simulink model "quadcopter_swarm_Perron"  (R2023b)
settings: Solver=ode3  StartTime=0  StopTime=inf  FixedStep=0.005  RelTol=1e-3  EnableMultiTasking=on
values from neighbouring files (symbols this model uses):
  F_e_g = [0 0 39.28]    [1nrx_dot.mat]    (also in 1nrxdrones_dot.mat; collision_avoidance_POS.mat; collision_avoidance_headonfix_POS.mat; collision_test.mat)
  g = 9.82    [1nrx_dot.mat]    (also in 1nrxdrones_dot.mat; collision_avoidance_POS.mat; collision_avoidance_headonfix_POS.mat; collision_test.mat)
  I_C = [0.5  0  0; 0  0.5  0; 0  0  1]    [1nrx_dot.mat]    (also in 1nrxdrones_dot.mat; collision_avoidance_POS.mat; collision_avoidance_headonfix_POS.mat; collision_test.mat)
  L = [4 -1 -1 -1 -1 0 -1 4 -1 -1 -1 0 ... (36 elements, 6x6)]    [1nrx_dot.mat]    (also in 1nrxdrones_dot.mat; collision_avoidance_POS.mat; collision_avoidance_headonfix_POS.mat; collision_test.mat)
  m = 4    [1nrx_dot.mat]    (also in 1nrxdrones_dot.mat; collision_avoidance_POS.mat; collision_avoidance_headonfix_POS.mat; collision_test.mat)
  M_RB = [4 0 0 0 0 0 0 4 0 0 0 0 ... (36 elements, 6x6)]    [1nrx_dot.mat]    (also in 1nrxdrones_dot.mat; collision_avoidance_POS.mat; collision_avoidance_headonfix_POS.mat; collision_test.mat)
  PID_inner_max = 100    [quadcopter_swarm_par.m]
  PID_outer_max = 10    [quadcopter_swarm_par.m]
  x_0 = [0, 3, 2, 1]'    [quadcopter_swarm_par.m]
  x_d = [1,4,-2,7]'    [quadcopter_swarm_par.m]
libraries: slpidlib x24, simulink_extras x20, dspsigops x12, aerolibutil x8, sharedtransform x4, vrlib x1
(part 1 of 5)
settings Model: Creator=The MathWorks, Inc.  LastModifiedBy=frank
settings SolverCC: AlgebraicLoopSolver=TrustRegion
settings DataIOCC: LimitDataPoints=on  SaveFormat=Array  SaveOutput=off  SignalLogging=off  DSMLogging=off  SaveTime=off  ReturnWorkspaceOutputs=off
settings OptimizationCC: BlockReduction=off  BufferReuse=off  LifeSpan=inf
settings DebuggingCC: AlgebraicLoopMsg=none  ParameterPrecisionLossMsg=none  AllowSymbolicDim=off  PregeneratedLibrarySubsystemCodeDiagnostic=none  SFUnexpectedBacktrackingDiag=warning  SFNoUnconditionalDefaultTransitionDiag=warning  SFExecutionAtInitializationDiag=none  ArithmeticOperatorsInVariantConditions=warning
settings HardwareCC: ProdBitPerPointer=32  ProdBitPerSizeT=32  ProdBitPerPtrDiffT=32  ProdLargestAtomicFloat=None  ProdIntDivRoundTo=Undefined  ProdEndianess=Unspecified  ProdWordSize=32  ProdHWDeviceType=32-bit Generic
settings ModelReferenceCC: EnableRefExpFcnMdlSchedulingChecks=on  PropagateSignalLabelsOutOfModel=off
settings SFSimCC: SimUseLocalCustomCode=off  CustomCodeUndefinedFunction=UseInterfaceOnly
settings RTWCC: RTWUseLocalCustomCode=off  DLArmComputeVersion=19.05
settings CodeAppCC: StateflowObjectComments=on
settings GRTTargetCC: TargetLangStandard=C89/C90 (ANSI)
settings ConfigComp: CovMetricSettings=dw  CovSaveCumulativeToWorkspaceVar=on  CovSaveSingleToWorkspaceVar=on  CovExternalEMLEnable=off  CovSFcnEnable=off

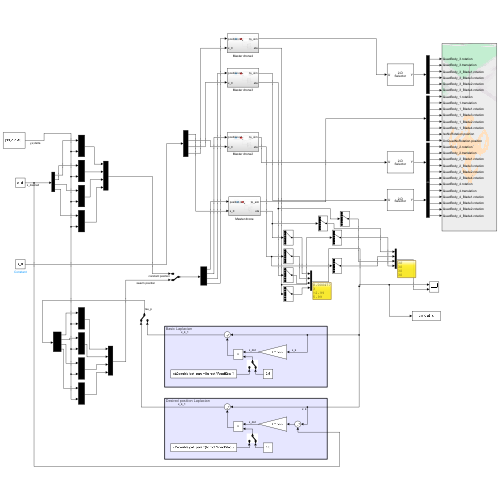
[thumbnail: Simulink's stored preview of the top-level diagram]
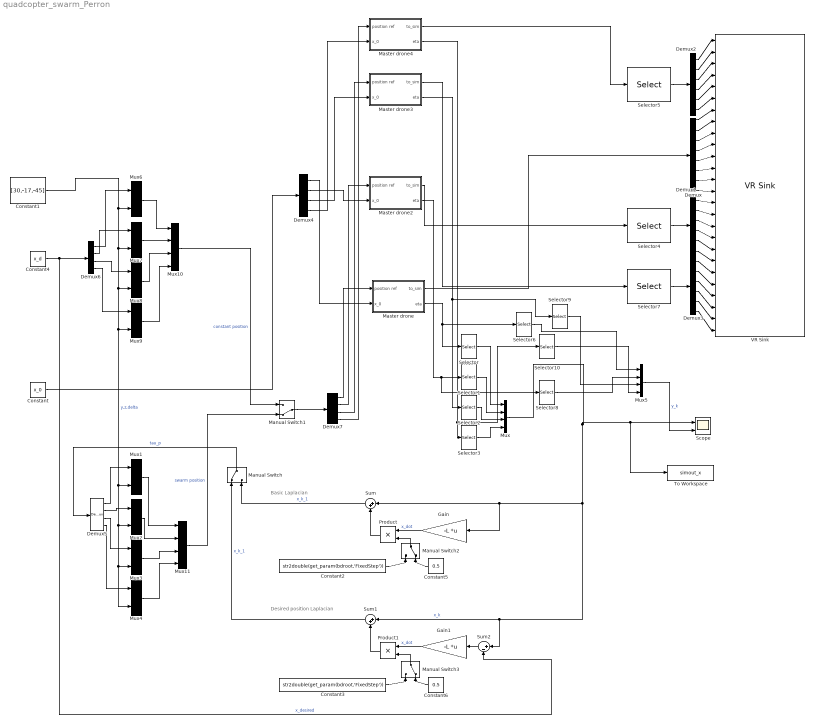
== system quadcopter_swarm_Perron ==
  note: Basic Laplacian
  note: Desired position Laplacian
  Constant : Constant  Value=x_0
  Constant1 : Constant  Value=[30,-17,-45]
  Constant2 : Constant  Value=str2double(get_param(bdroot,'FixedStep'))
  Constant3 : Constant  Value=str2double(get_param(bdroot,'FixedStep'))
  Constant4 : Constant  Value=x_d
  Constant5 : Constant  Value=0.5
  Constant6 : Constant  Value=0.5
  Demux : Demux  Outputs=8
  Demux1 : Demux  Outputs=6
  Demux2 : Demux  Outputs=6
  Demux3 : Demux  Outputs=6
  Demux{4..7} (4 alike) : Demux
  Gain : Gain  Gain=-L  Multiplication=Matrix(K*u) (u vector)
  Gain1 : Gain  Gain=-L  Multiplication=Matrix(K*u) (u vector)
  Manual Switch : ManualSwitch
  Manual Switch1 : ManualSwitch  CurrentSetting=0
  Manual Switch2 : ManualSwitch  CurrentSetting=0
  Manual Switch3 : ManualSwitch  CurrentSetting=0
  Master drone : Subsystem
  Master drone2 : Subsystem
  Master drone3 : Subsystem
  Master drone4 : Subsystem
  Mux{,5,10..11} (4 alike) : Mux
  Mux{1..4,6..9} (8 alike) : Mux  Inputs=2
  Product : Product
  Product1 : Product
  Scope : Scope  NumInputPorts=2
  Selector{,1..3} (4 alike) : Selector  InputPortWidth=6  IndexOptions=Index vector (dialog)  Indices=1  OutputSizes=1
  Selector{6,8..10} (4 alike) : Selector  InputPortWidth=6  IndexOptions=Index vector (dialog)  Indices=2  OutputSizes=1
  Selector4 : Selector  NumberOfDimensions=2  InputPortWidth=8  IndexOptions=Index vector (dialog),Select all  Indices=1:23,1  OutputSizes=1,1
  Selector5 : Selector  NumberOfDimensions=2  InputPortWidth=8  IndexOptions=Index vector (dialog),Select all  Indices=1:23,1  OutputSizes=1,1
  Selector7 : Selector  NumberOfDimensions=2  InputPortWidth=8  IndexOptions=Index vector (dialog),Select all  Indices=1:23,1  OutputSizes=1,1
  Sum : Sum  Inputs=|++
  Sum1 : Sum  Inputs=|++
  Sum2 : Sum  Inputs=|+-
  To Workspace : ToWorkspace  VariableName=simout_x  SampleTime=-1
      settings: Save2DSignal=2-D array (concatenate along first dimension)
  VR Sink : vrlib/VR Sink  InstantiateOnLoad=on  SampleTime=12*0.005  ViewEnable=on  RemoteChange=off  RemoteView=off  FieldsWritten=QuadBody_3.rotation.4.1.1.double#QuadBody_3.translation.3.1.1.double#QuadBody_3_Blade1.rotation.4.1.1.double#QuadBody_3_Blade3.rotation.4.1.1.double#QuadBody_3_Blade2.rotation.4.1.1.double#QuadBody_3_Blade4.rotation.4.1.1.double#QuadBody_1.rotation.4.1.1.double#QuadBody_1.translation.3.1.1.double#QuadBody_1_Blade1.rotation.4.1.1.double#QuadBody_1_Blade3.rotation.4.1.1.double#QuadBody_1_Blade2.rotation.4.1.1.double#QuadBody_1_Blade4.rotation.4.1.1.double#IsoNoRotation.position.3.1.1.double#OnQuadNoRotation.position.3.1.1.double#QuadBody_2.rotation.4.1.1.double#QuadBody_2.translation.3.1.1.double#QuadBody_2_Blade1.rotation.4.1.1.double#QuadBody_2_Blade3.rotation.4.1.1.double#QuadBody_2_Blade2.rotation.4.1.1.double#QuadBody_2_Blade4.rotation.4.1.1.double#QuadBody_4.rotation.4.1.1.double#QuadBody_4.translation.3.1.1.double#QuadBody_4_Blade1.rotation.4.1.1.double#QuadBody_4_Blade3.rotation.4.1.1.double#QuadBody_4_Blade2.rotation.4.1.1.double#QuadBody_4_Blade4.rotation.4.1.1.double  WorldFileName=Quadcopter_VR.wrl  AutoView=on  VideoDimensions=[]  AllowVariableSize=off  FigureProperties="{'Position', 'Name', 'Viewpoint', 'CameraBound', 'CameraDirection', 'CameraPosition', 'CameraUpVector', 'ZoomFactor', 'Antialiasing', 'Headlight', 'Lighting', 'NavPanel', 'Sound', 'StatusBar', 'Stereo3D', 'Stereo3DCameraOffset', 'Stereo3DHIT', 'ToolBar', 'Textures', 'Transparency', 'Triad', 'Wireframe', 'NavZones', 'NavMode', 'NavSpeed', 'CaptureFileFormat', 'CaptureFileName', 'Record2DCompressMethod', 'Record2DCompressQuality', 'Record2D', 'Record2DFileName', 'Record2DFPS'; [4.4020000000000000e+03   4.4400000000000000e+02   9.5800000000000000e+02   9.0400000000000000e+02], '', 'Isometric - No Rotation', 'on', [6.2775029607530120e-02  -3.1395260637159403e-02  -9.9753377550201194e-01], [0.0000000000000000e+00   0.0000000000000000e+00   1.5000000000000000e+01], [9.8663584075743787e-04   9.9950656033827134e-01  -3.1395260637159403e-02], [1.0000000000000000e+00], 'on', 'on', 'on', 'halfbar', 'on', 'on', 'off', [1.0000000149011612e-01], [0.0000000000000000e+00], 'on', 'on', 'on', 'none', 'off', 'off', 'fly', 'normal', 'tif', '%f_anim_%n.tif', 'auto', [7.5000000000000000e+01], 'off', '%f_anim_%n.avi', 'auto'}"
  wires:
  Demux/1 -> VR Sink/7
  Demux/2 -> VR Sink/8
  Demux/3 -> VR Sink/9
  Demux/4 -> VR Sink/10
  Demux/5 -> VR Sink/11
  Demux/6 -> VR Sink/12
  Demux1/1 -> VR Sink/15
  Demux1/2 -> VR Sink/16
  Demux1/3 -> VR Sink/17
  Demux1/4 -> VR Sink/18
  Demux1/5 -> VR Sink/19
  Demux1/6 -> VR Sink/20
  Demux3/1 -> VR Sink/21
  Demux3/2 -> VR Sink/22
  Demux3/3 -> VR Sink/23
  Demux3/4 -> VR Sink/24
  Demux3/5 -> VR Sink/25
  Demux3/6 -> VR Sink/26
  Demux2/6 -> VR Sink/6
  Demux2/5 -> VR Sink/5
  Demux2/4 -> VR Sink/4
  Demux2/3 -> VR Sink/3
  Demux2/2 -> VR Sink/2
  Demux2/1 -> VR Sink/1
  Selector5/1 -> Demux2/1
  Selector7/1 -> Demux3/1
  Master drone4/1(to_sim) -> Selector5/1
  Selector4/1 -> Demux1/1
  Demux/7 -> VR Sink/13
  Demux/8 -> VR Sink/14
  Master drone/1(to_sim) -> Demux/1
  Master drone2/1(to_sim) -> Selector4/1
  Master drone3/1(to_sim) -> Selector7/1
  Master drone/2(eta) -> Selector/1, Selector6/1
  Master drone2/2(eta) -> Selector8/1, Selector1/1
  Master drone3/2(eta) -> Selector2/1, Selector9/1
  Master drone4/2(eta) -> Selector3/1, Selector10/1
  Selector/1 -> Mux/1
  Selector1/1 -> Mux/2
  Selector2/1 -> Mux/3
  Selector3/1 -> Mux/4
  Constant/1 -> Demux4/1
  Demux4/1 -> Master drone/2(x_0)
  Demux4/2 -> Master drone2/2(x_0)
  Demux4/3 -> Master drone3/2(x_0)
  Demux4/4 -> Master drone4/2(x_0)
  Sum/1 -> Manual Switch/2  "x_k_1"
  Demux7/1 -> Master drone/1(position ref)
  Demux5/1 -> Mux1/1
  Demux5/2 -> Mux2/1
  Demux7/2 -> Master drone2/1(position ref)
  Demux5/3 -> Mux3/1
  Demux5/4 -> Mux4/1
  Demux7/3 -> Master drone3/1(position ref)
  Demux7/4 -> Master drone4/1(position ref)
  Selector6/1 -> Mux5/1
  Selector8/1 -> Mux5/2
  Selector9/1 -> Mux5/3
  Selector10/1 -> Mux5/4
  Mux5/1 -> Scope/2  "y_k"
  Gain/1 -> Product/1  "x_dot"
  Constant2/1 -> Manual Switch2/1
  Product/1 -> Sum/2
  Product1/1 -> Sum1/2
  Sum1/1 -> Manual Switch/1  "x_k_1"
  Gain1/1 -> Product1/1  "x_dot"
  Mux/1 -> Sum2/1, Sum1/1, Sum/1, Gain/1, To Workspace/1, Scope/1  "x_k"
  Manual Switch/1 -> Demux5/1  "tau_p"
  Constant1/1 -> Mux4/2, Mux3/2, Mux2/2, Mux1/2, Mux9/2, Mux8/2, Mux7/2, Mux6/2  "y,z,delta"
  Mux6/1 -> Mux10/1
  Mux7/1 -> Mux10/2
  Mux8/1 -> Mux10/3
  Mux9/1 -> Mux10/4
  Manual Switch1/1 -> Demux7/1
  Mux11/1 -> Manual Switch1/2  "swarm position"
  Mux10/1 -> Manual Switch1/1  "constant position"
  Mux1/1 -> Mux11/1
  Mux2/1 -> Mux11/2
  Mux3/1 -> Mux11/3
  Mux4/1 -> Mux11/4
  Constant4/1 -> Sum2/2, Demux6/1  "x_desired"
  Demux6/1 -> Mux6/1
  Demux6/2 -> Mux7/1
  Demux6/3 -> Mux8/1
  Demux6/4 -> Mux9/1
  Constant5/1 -> Manual Switch2/2
  Manual Switch2/1 -> Product/2
  Sum2/1 -> Gain1/1
  Constant6/1 -> Manual Switch3/2
  Constant3/1 -> Manual Switch3/1
  Manual Switch3/1 -> Product1/2

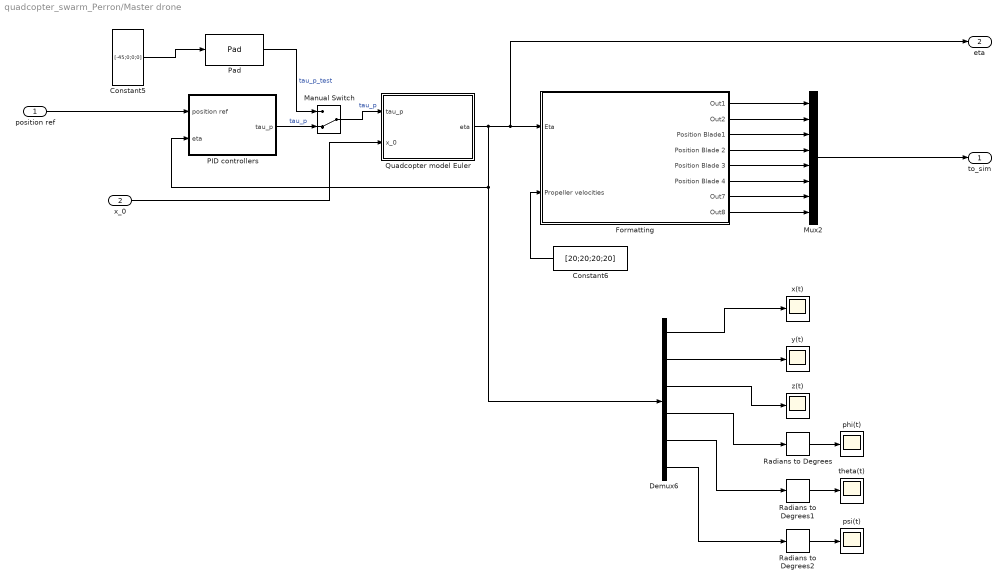
== system quadcopter_swarm_Perron/Master drone ==
  position ref : Inport
  x_0 : Inport  Port=2
  Constant5 : Constant  Value=[-45;0;0;0]  VectorParams1D=off
  Constant6 : Constant  Value=[20;20;20;20]  VectorParams1D=off
  Demux6 : Demux  Outputs=6
  Formatting : Subsystem
  Manual Switch : ManualSwitch  CurrentSetting=0
  Mux2 : Mux  Inputs=8
  PID controllers : Subsystem
  Pad : dspsigops/Pad  padAlong=Specified dimensions  dimsToPad=1  valSrc=Specify via dialog  padVal=0  spec=Output size  padNumOutRowsSpecMethod=User-specified  numOutRows=1  padNumOutColsSpecMethod=User-specified  numOutCols=6  isVarDimsMode=off  padBeginning=0  padEnd=0  outSizeMode=User-specified  outSize=6  padSigAt=Beginning  trunc_flag=None  roundingMode=Floor  overflowMode=off  truncOrWrapMode=Truncate  wrap_flag=None
  Quadcopter model Euler : Subsystem
  Radians to Degrees : simulink_extras/Transformations/Radians to Degrees
  Radians to Degrees1 : simulink_extras/Transformations/Radians to Degrees
  Radians to Degrees2 : simulink_extras/Transformations/Radians to Degrees
  phi(t) : Scope
  psi(t) : Scope
  theta(t) : Scope
  x(t) : Scope
  y(t) : Scope
  z(t) : Scope
  to_sim : Outport
  eta : Outport  Port=2
  wires:
  Formatting/6(Position Blade 4) -> Mux2/6
  Demux6/1 -> x(t)/1
  Demux6/6 -> Radians to Degrees2/1
  Manual Switch/1 -> Quadcopter model Euler/1(tau_p)  "tau_p"
  Pad/1 -> Manual Switch/1  "tau_p_test"
  Radians to Degrees2/1 -> psi(t)/1
  Demux6/5 -> Radians to Degrees1/1
  Formatting/3(Position Blade1) -> Mux2/3
  Formatting/2(Out2) -> Mux2/2
  Demux6/4 -> Radians to Degrees/1
  position ref/1 -> PID controllers/1(position ref)
  Demux6/3 -> z(t)/1
  Constant6/1 -> Formatting/2(Propeller velocities)
  Constant5/1 -> Pad/1
  Demux6/2 -> y(t)/1
  Formatting/7(Out7) -> Mux2/7
  Radians to Degrees1/1 -> theta(t)/1
  Formatting/8(Out8) -> Mux2/8
  Radians to Degrees/1 -> phi(t)/1
  Formatting/5(Position Blade 3) -> Mux2/5
  Formatting/4(Position Blade 2) -> Mux2/4
  Formatting/1(Out1) -> Mux2/1
  PID controllers/1(tau_p) -> Manual Switch/2  "tau_p"
  Mux2/1 -> to_sim/1
  Quadcopter model Euler/1(eta) -> Demux6/1, PID controllers/2(eta), eta/1, Formatting/1(Eta)
  x_0/1 -> Quadcopter model Euler/2(x_0)

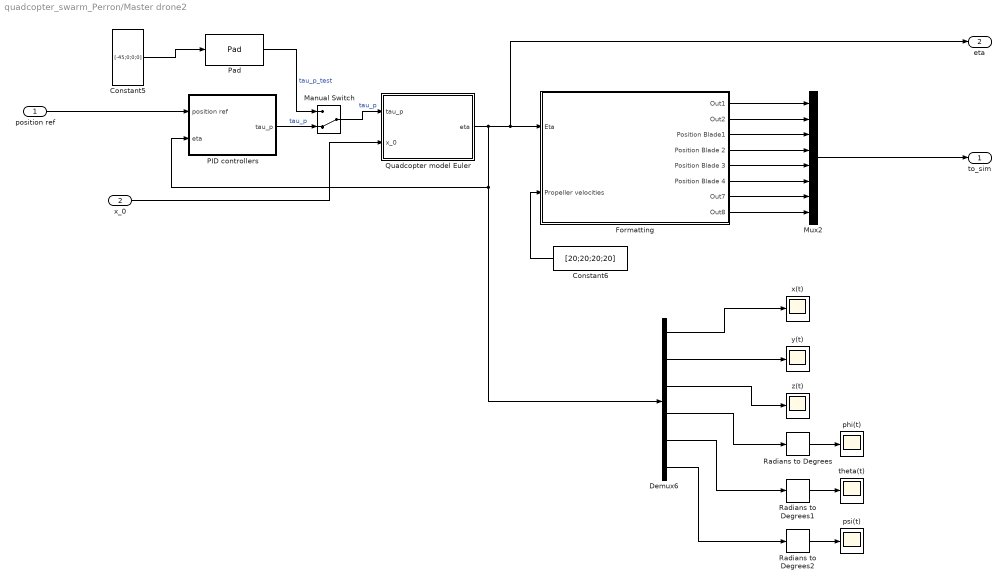
== system quadcopter_swarm_Perron/Master drone2 ==
  position ref : Inport
  x_0 : Inport  Port=2
  Constant5 : Constant  Value=[-45;0;0;0]  VectorParams1D=off
  Constant6 : Constant  Value=[20;20;20;20]  VectorParams1D=off
  Demux6 : Demux  Outputs=6
  Formatting : Subsystem
  Manual Switch : ManualSwitch  CurrentSetting=0
  Mux2 : Mux  Inputs=8
  PID controllers : Subsystem
  Pad : dspsigops/Pad  padAlong=Specified dimensions  dimsToPad=1  valSrc=Specify via dialog  padVal=0  spec=Output size  padNumOutRowsSpecMethod=User-specified  numOutRows=1  padNumOutColsSpecMethod=User-specified  numOutCols=6  isVarDimsMode=off  padBeginning=0  padEnd=0  outSizeMode=User-specified  outSize=6  padSigAt=Beginning  trunc_flag=None  roundingMode=Floor  overflowMode=off  truncOrWrapMode=Truncate  wrap_flag=None
  Quadcopter model Euler : Subsystem
  Radians to Degrees : simulink_extras/Transformations/Radians to Degrees
  Radians to Degrees1 : simulink_extras/Transformations/Radians to Degrees
  Radians to Degrees2 : simulink_extras/Transformations/Radians to Degrees
  phi(t) : Scope
  psi(t) : Scope
  theta(t) : Scope
  x(t) : Scope
  y(t) : Scope
  z(t) : Scope
  to_sim : Outport
  eta : Outport  Port=2
  wires:
  Formatting/6(Position Blade 4) -> Mux2/6
  Demux6/1 -> x(t)/1
  Demux6/6 -> Radians to Degrees2/1
  Manual Switch/1 -> Quadcopter model Euler/1(tau_p)  "tau_p"
  Pad/1 -> Manual Switch/1  "tau_p_test"
  Radians to Degrees2/1 -> psi(t)/1
  Demux6/5 -> Radians to Degrees1/1
  Formatting/3(Position Blade1) -> Mux2/3
  Formatting/2(Out2) -> Mux2/2
  Demux6/4 -> Radians to Degrees/1
  position ref/1 -> PID controllers/1(position ref)
  Demux6/3 -> z(t)/1
  Constant6/1 -> Formatting/2(Propeller velocities)
  Constant5/1 -> Pad/1
  Demux6/2 -> y(t)/1
  Formatting/7(Out7) -> Mux2/7
  Radians to Degrees1/1 -> theta(t)/1
  Formatting/8(Out8) -> Mux2/8
  Radians to Degrees/1 -> phi(t)/1
  Formatting/5(Position Blade 3) -> Mux2/5
  Formatting/4(Position Blade 2) -> Mux2/4
  Formatting/1(Out1) -> Mux2/1
  PID controllers/1(tau_p) -> Manual Switch/2  "tau_p"
  Mux2/1 -> to_sim/1
  Quadcopter model Euler/1(eta) -> Demux6/1, PID controllers/2(eta), eta/1, Formatting/1(Eta)
  x_0/1 -> Quadcopter model Euler/2(x_0)

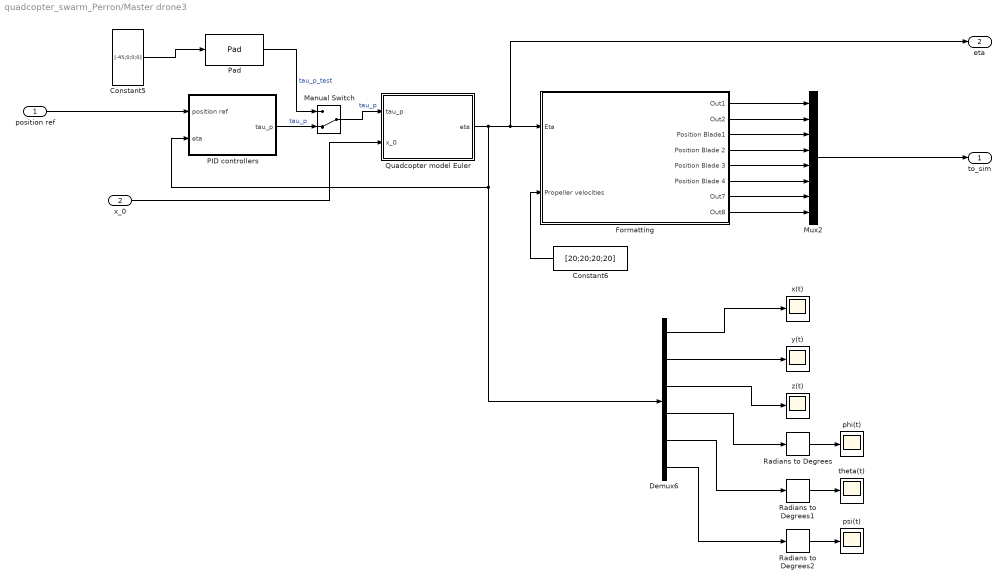
== system quadcopter_swarm_Perron/Master drone3 ==
  position ref : Inport
  x_0 : Inport  Port=2
  Constant5 : Constant  Value=[-45;0;0;0]  VectorParams1D=off
  Constant6 : Constant  Value=[20;20;20;20]  VectorParams1D=off
  Demux6 : Demux  Outputs=6
  Formatting : Subsystem
  Manual Switch : ManualSwitch  CurrentSetting=0
  Mux2 : Mux  Inputs=8
  PID controllers : Subsystem
  Pad : dspsigops/Pad  padAlong=Specified dimensions  dimsToPad=1  valSrc=Specify via dialog  padVal=0  spec=Output size  padNumOutRowsSpecMethod=User-specified  numOutRows=1  padNumOutColsSpecMethod=User-specified  numOutCols=6  isVarDimsMode=off  padBeginning=0  padEnd=0  outSizeMode=User-specified  outSize=6  padSigAt=Beginning  trunc_flag=None  roundingMode=Floor  overflowMode=off  truncOrWrapMode=Truncate  wrap_flag=None
  Quadcopter model Euler : Subsystem
  Radians to Degrees : simulink_extras/Transformations/Radians to Degrees
  Radians to Degrees1 : simulink_extras/Transformations/Radians to Degrees
  Radians to Degrees2 : simulink_extras/Transformations/Radians to Degrees
  phi(t) : Scope
  psi(t) : Scope
  theta(t) : Scope
  x(t) : Scope
  y(t) : Scope
  z(t) : Scope
  to_sim : Outport
  eta : Outport  Port=2
  wires:
  Formatting/6(Position Blade 4) -> Mux2/6
  Demux6/1 -> x(t)/1
  Demux6/6 -> Radians to Degrees2/1
  Manual Switch/1 -> Quadcopter model Euler/1(tau_p)  "tau_p"
  Pad/1 -> Manual Switch/1  "tau_p_test"
  Radians to Degrees2/1 -> psi(t)/1
  Demux6/5 -> Radians to Degrees1/1
  Formatting/3(Position Blade1) -> Mux2/3
  Formatting/2(Out2) -> Mux2/2
  Demux6/4 -> Radians to Degrees/1
  position ref/1 -> PID controllers/1(position ref)
  Demux6/3 -> z(t)/1
  Constant6/1 -> Formatting/2(Propeller velocities)
  Constant5/1 -> Pad/1
  Demux6/2 -> y(t)/1
  Formatting/7(Out7) -> Mux2/7
  Radians to Degrees1/1 -> theta(t)/1
  Formatting/8(Out8) -> Mux2/8
  Radians to Degrees/1 -> phi(t)/1
  Formatting/5(Position Blade 3) -> Mux2/5
  Formatting/4(Position Blade 2) -> Mux2/4
  Formatting/1(Out1) -> Mux2/1
  PID controllers/1(tau_p) -> Manual Switch/2  "tau_p"
  Mux2/1 -> to_sim/1
  Quadcopter model Euler/1(eta) -> Demux6/1, PID controllers/2(eta), eta/1, Formatting/1(Eta)
  x_0/1 -> Quadcopter model Euler/2(x_0)

== system quadcopter_swarm_Perron/Master drone4 ==
  position ref : Inport
  x_0 : Inport  Port=2
  Constant5 : Constant  Value=[-45;0;0;0]  VectorParams1D=off
  Constant6 : Constant  Value=[20;20;20;20]  VectorParams1D=off
  Demux6 : Demux  Outputs=6
  Formatting : Subsystem
  Manual Switch : ManualSwitch  CurrentSetting=0
  Mux2 : Mux  Inputs=8
  PID controllers : Subsystem
  Pad : dspsigops/Pad  padAlong=Specified dimensions  dimsToPad=1  valSrc=Specify via dialog  padVal=0  spec=Output size  padNumOutRowsSpecMethod=User-specified  numOutRows=1  padNumOutColsSpecMethod=User-specified  numOutCols=6  isVarDimsMode=off  padBeginning=0  padEnd=0  outSizeMode=User-specified  outSize=6  padSigAt=Beginning  trunc_flag=None  roundingMode=Floor  overflowMode=off  truncOrWrapMode=Truncate  wrap_flag=None
  Quadcopter model Euler : Subsystem
  Radians to Degrees : simulink_extras/Transformations/Radians to Degrees
  Radians to Degrees1 : simulink_extras/Transformations/Radians to Degrees
  Radians to Degrees2 : simulink_extras/Transformations/Radians to Degrees
  phi(t) : Scope
  psi(t) : Scope
  theta(t) : Scope
  x(t) : Scope
  y(t) : Scope
  z(t) : Scope
  to_sim : Outport
  eta : Outport  Port=2
  wires:
  Formatting/6(Position Blade 4) -> Mux2/6
  Demux6/1 -> x(t)/1
  Demux6/6 -> Radians to Degrees2/1
  Manual Switch/1 -> Quadcopter model Euler/1(tau_p)  "tau_p"
  Pad/1 -> Manual Switch/1  "tau_p_test"
  Radians to Degrees2/1 -> psi(t)/1
  Demux6/5 -> Radians to Degrees1/1
  Formatting/3(Position Blade1) -> Mux2/3
  Formatting/2(Out2) -> Mux2/2
  Demux6/4 -> Radians to Degrees/1
  position ref/1 -> PID controllers/1(position ref)
  Demux6/3 -> z(t)/1
  Constant6/1 -> Formatting/2(Propeller velocities)
  Constant5/1 -> Pad/1
  Demux6/2 -> y(t)/1
  Formatting/7(Out7) -> Mux2/7
  Radians to Degrees1/1 -> theta(t)/1
  Formatting/8(Out8) -> Mux2/8
  Radians to Degrees/1 -> phi(t)/1
  Formatting/5(Position Blade 3) -> Mux2/5
  Formatting/4(Position Blade 2) -> Mux2/4
  Formatting/1(Out1) -> Mux2/1
  PID controllers/1(tau_p) -> Manual Switch/2  "tau_p"
  Mux2/1 -> to_sim/1
  Quadcopter model Euler/1(eta) -> Demux6/1, PID controllers/2(eta), eta/1, Formatting/1(Eta)
  x_0/1 -> Quadcopter model Euler/2(x_0)

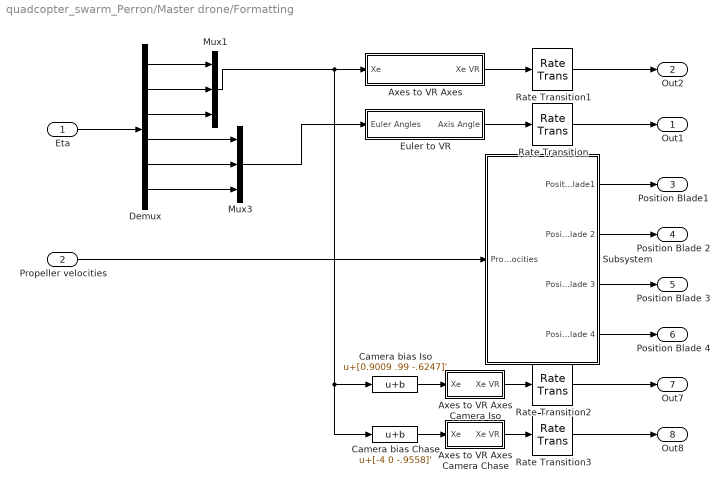
== system quadcopter_swarm_Perron/Master drone/Formatting ==
  Eta : Inport
  Propeller velocities : Inport  Port=2
  Axes to VR Axes : Subsystem
  Axes to VR Axes Camera Chase : Subsystem
  Axes to VR Axes Camera Iso : Subsystem
  Camera bias Chase : Bias  Bias=[-4 0 -.9558]'  SaturateOnIntegerOverflow=off
  Camera bias Iso : Bias  Bias=[0.9009 .99 -.6247]'  SaturateOnIntegerOverflow=off
  Demux : Demux  Outputs=6
  Euler to VR : Subsystem
  Mux1 : Mux  Inputs=3
  Mux3 : Mux  Inputs=3
  Rate Transition{,1..3} (4 alike) : RateTransition
  Subsystem : Subsystem
  Out1 : Outport
  Out2 : Outport  Port=2
  Position Blade1 : Outport  Port=3
  Position Blade 2 : Outport  Port=4
  Position Blade 3 : Outport  Port=5
  Position Blade 4 : Outport  Port=6
  Out7 : Outport  Port=7
  Out8 : Outport  Port=8
  wires:
  Rate Transition2/1 -> Out7/1
  Propeller velocities/1 -> Subsystem/1(Propeller velocities)
  Subsystem/3(Position Blade 3) -> Position Blade 3/1
  Subsystem/1(Position Blade1) -> Position Blade1/1
  Mux3/1 -> Euler to VR/1(Euler Angles)
  Camera bias Chase/1 -> Axes to VR Axes Camera Chase/1(Xe)
  Axes to VR Axes Camera Chase/1(Xe VR) -> Rate Transition3/1
  Subsystem/2(Position Blade 2) -> Position Blade 2/1
  Axes to VR Axes Camera Iso/1(Xe VR) -> Rate Transition2/1
  Euler to VR/1(Axis Angle) -> Rate Transition/1
  Axes to VR Axes/1(Xe VR) -> Rate Transition1/1
  Rate Transition1/1 -> Out2/1
  Camera bias Iso/1 -> Axes to VR Axes Camera Iso/1(Xe)
  Mux1/1 -> Camera bias Chase/1, Camera bias Iso/1, Axes to VR Axes/1(Xe)
  Rate Transition3/1 -> Out8/1
  Rate Transition/1 -> Out1/1
  Subsystem/4(Position Blade 4) -> Position Blade 4/1
  Demux/2 -> Mux1/2
  Demux/5 -> Mux3/2
  Demux/3 -> Mux1/3
  Eta/1 -> Demux/1
  Demux/1 -> Mux1/1
  Demux/4 -> Mux3/1
  Demux/6 -> Mux3/3

== system quadcopter_swarm_Perron/Master drone/PID controllers ==
  position ref : Inport
  eta : Inport  Port=2
  Inner-loop controllers : Subsystem
  Manual Switch : ManualSwitch
  Pad3 : dspsigops/Pad  padAlong=Rows  dimsToPad=1  valSrc=Specify via dialog  padVal=0  spec=Output size  padNumOutRowsSpecMethod=User-specified  numOutRows=1  padNumOutColsSpecMethod=User-specified  numOutCols=6  isVarDimsMode=off  padBeginning=0  padEnd=0  outSizeMode=User-specified  outSize=1  padSigAt=Beginning  trunc_flag=None  roundingMode=Floor  overflowMode=off  truncOrWrapMode=Truncate  wrap_flag=None
  Refs (alt. + Euler angles) : Constant  Value=[-20;0;20;0]  VectorParams1D=off
  outer-loop controllers output : Scope
  outer-loop position controller : Subsystem
  tau_p : Outport
  wires:
  position ref/1 -> outer-loop position controller/1(position ref)
  outer-loop position controller/1(alt. + Euler angles) -> Manual Switch/1, outer-loop controllers output/1
  eta/1 -> Inner-loop controllers/2(eta), outer-loop position controller/2(eta_euler)  "eta_euler"
  Refs (alt. + Euler angles)/1 -> Manual Switch/2
  Manual Switch/1 -> Inner-loop controllers/1(refs)  "alt. + Euler angles"
  Pad3/1 -> tau_p/1
  Inner-loop controllers/1(Fz,mx,my,mz) -> Pad3/1

== system quadcopter_swarm_Perron/Master drone/Quadcopter model Euler ==
  tau_p : Inport
  x_0 : Inport  Port=2
  Gravity : Subsystem
      settings: PortSchema="{\"entries\":[{\"content\":{\"sides\":[{\"content\":{\"connectorIds\":[\"Out1\",\"In1\"]},\"type\":\"ConnectorPlacement.EquallySpacedRectSide\",\"uuid\":\"bc23a1f5-cdb9-4283-9ea4-cdee480fdcbc\"},{\"content\":{\"side\":\"RIGHT\"},\"type\":\"ConnectorPlacement.EquallySpacedRectSide\",\"uuid\":\"6d80009b-5037-4ff5-9c53-c950dec4dc37\"},{\"content\":{\"side\":\"TOP\"},\"type\":\"ConnectorPlacement.EquallySpacedRectSide\",\"uuid\":\"00364382-26ff-4cd9-a2a2-07aec872e2b0\"}]},\"type\":\"ConnectorPlacement.EquallySpacedConnector\",\"uuid\":\"88fcb791-5b95-44c0-bf21-2ced4fb8e0fb\"}],\"packageUris\":[\"http://schema.mathworks.com/mf0/Connector/R2020b\"],\"version\":\"1.0\"}"
  Scope1 : Scope  NumInputPorts=3
  Sum : Sum  Inputs=|++
  kinematics from Euler angles : Subsystem
  rigid-body dynamics : Subsystem
  eta : Outport
  wires:
  kinematics from Euler angles/1(eta) -> eta/1, Gravity/1(eta_euler), Scope1/3
  tau_p/1 -> Sum/1  "tau_p"
  Sum/1 -> Scope1/1, rigid-body dynamics/1(tau)  "tau"
  rigid-body dynamics/1(nu_subsystem) -> Scope1/2, kinematics from Euler angles/1(nu)
  Gravity/1(tau_g) -> Sum/2
  x_0/1 -> kinematics from Euler angles/2(x_0)

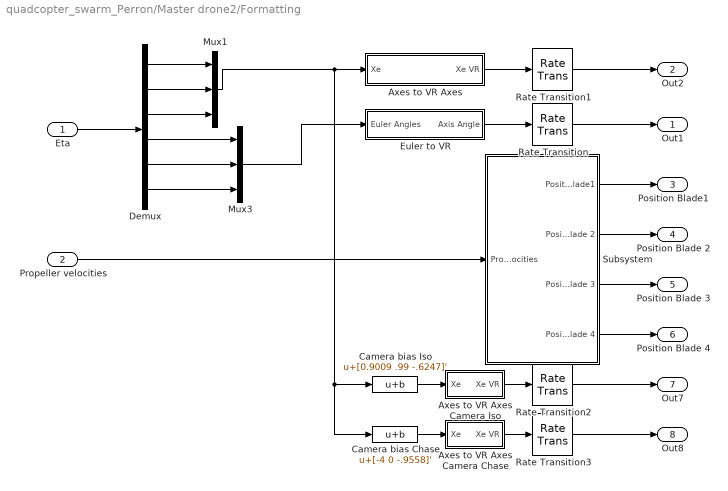
== system quadcopter_swarm_Perron/Master drone2/Formatting ==
  Eta : Inport
  Propeller velocities : Inport  Port=2
  Axes to VR Axes : Subsystem
  Axes to VR Axes Camera Chase : Subsystem
  Axes to VR Axes Camera Iso : Subsystem
  Camera bias Chase : Bias  Bias=[-4 0 -.9558]'  SaturateOnIntegerOverflow=off
  Camera bias Iso : Bias  Bias=[0.9009 .99 -.6247]'  SaturateOnIntegerOverflow=off
  Demux : Demux  Outputs=6
  Euler to VR : Subsystem
  Mux1 : Mux  Inputs=3
  Mux3 : Mux  Inputs=3
  Rate Transition{,1..3} (4 alike) : RateTransition
  Subsystem : Subsystem
  Out1 : Outport
  Out2 : Outport  Port=2
  Position Blade1 : Outport  Port=3
  Position Blade 2 : Outport  Port=4
  Position Blade 3 : Outport  Port=5
  Position Blade 4 : Outport  Port=6
  Out7 : Outport  Port=7
  Out8 : Outport  Port=8
  wires:
  Rate Transition2/1 -> Out7/1
  Propeller velocities/1 -> Subsystem/1(Propeller velocities)
  Subsystem/3(Position Blade 3) -> Position Blade 3/1
  Subsystem/1(Position Blade1) -> Position Blade1/1
  Mux3/1 -> Euler to VR/1(Euler Angles)
  Camera bias Chase/1 -> Axes to VR Axes Camera Chase/1(Xe)
  Axes to VR Axes Camera Chase/1(Xe VR) -> Rate Transition3/1
  Subsystem/2(Position Blade 2) -> Position Blade 2/1
  Axes to VR Axes Camera Iso/1(Xe VR) -> Rate Transition2/1
  Euler to VR/1(Axis Angle) -> Rate Transition/1
  Axes to VR Axes/1(Xe VR) -> Rate Transition1/1
  Rate Transition1/1 -> Out2/1
  Camera bias Iso/1 -> Axes to VR Axes Camera Iso/1(Xe)
  Mux1/1 -> Camera bias Chase/1, Camera bias Iso/1, Axes to VR Axes/1(Xe)
  Rate Transition3/1 -> Out8/1
  Rate Transition/1 -> Out1/1
  Subsystem/4(Position Blade 4) -> Position Blade 4/1
  Demux/2 -> Mux1/2
  Demux/5 -> Mux3/2
  Demux/3 -> Mux1/3
  Eta/1 -> Demux/1
  Demux/1 -> Mux1/1
  Demux/4 -> Mux3/1
  Demux/6 -> Mux3/3

== system quadcopter_swarm_Perron/Master drone2/PID controllers ==
  position ref : Inport
  eta : Inport  Port=2
  Inner-loop controllers : Subsystem
  Manual Switch : ManualSwitch
  Pad3 : dspsigops/Pad  padAlong=Rows  dimsToPad=1  valSrc=Specify via dialog  padVal=0  spec=Output size  padNumOutRowsSpecMethod=User-specified  numOutRows=1  padNumOutColsSpecMethod=User-specified  numOutCols=6  isVarDimsMode=off  padBeginning=0  padEnd=0  outSizeMode=User-specified  outSize=1  padSigAt=Beginning  trunc_flag=None  roundingMode=Floor  overflowMode=off  truncOrWrapMode=Truncate  wrap_flag=None
  Refs (alt. + Euler angles) : Constant  Value=[-20;0;20;0]  VectorParams1D=off
  outer-loop controllers output : Scope
  outer-loop position controller : Subsystem
  tau_p : Outport
  wires:
  position ref/1 -> outer-loop position controller/1(position ref)
  outer-loop position controller/1(alt. + Euler angles) -> Manual Switch/1, outer-loop controllers output/1
  eta/1 -> Inner-loop controllers/2(eta), outer-loop position controller/2(eta_euler)  "eta_euler"
  Refs (alt. + Euler angles)/1 -> Manual Switch/2
  Manual Switch/1 -> Inner-loop controllers/1(refs)  "alt. + Euler angles"
  Pad3/1 -> tau_p/1
  Inner-loop controllers/1(Fz,mx,my,mz) -> Pad3/1

== system quadcopter_swarm_Perron/Master drone2/Quadcopter model Euler ==
  tau_p : Inport
  x_0 : Inport  Port=2
  Gravity : Subsystem
      settings: PortSchema="{\"entries\":[{\"content\":{\"sides\":[{\"content\":{\"connectorIds\":[\"Out1\",\"In1\"]},\"type\":\"ConnectorPlacement.EquallySpacedRectSide\",\"uuid\":\"bc23a1f5-cdb9-4283-9ea4-cdee480fdcbc\"},{\"content\":{\"side\":\"RIGHT\"},\"type\":\"ConnectorPlacement.EquallySpacedRectSide\",\"uuid\":\"6d80009b-5037-4ff5-9c53-c950dec4dc37\"},{\"content\":{\"side\":\"TOP\"},\"type\":\"ConnectorPlacement.EquallySpacedRectSide\",\"uuid\":\"00364382-26ff-4cd9-a2a2-07aec872e2b0\"}]},\"type\":\"ConnectorPlacement.EquallySpacedConnector\",\"uuid\":\"88fcb791-5b95-44c0-bf21-2ced4fb8e0fb\"}],\"packageUris\":[\"http://schema.mathworks.com/mf0/Connector/R2020b\"],\"version\":\"1.0\"}"
  Scope1 : Scope  NumInputPorts=3
  Sum : Sum  Inputs=|++
  kinematics from Euler angles : Subsystem
  rigid-body dynamics : Subsystem
  eta : Outport
  wires:
  kinematics from Euler angles/1(eta) -> eta/1, Gravity/1(eta_euler), Scope1/3
  tau_p/1 -> Sum/1  "tau_p"
  Sum/1 -> Scope1/1, rigid-body dynamics/1(tau)  "tau"
  rigid-body dynamics/1(nu_subsystem) -> Scope1/2, kinematics from Euler angles/1(nu)
  Gravity/1(tau_g) -> Sum/2
  x_0/1 -> kinematics from Euler angles/2(x_0)

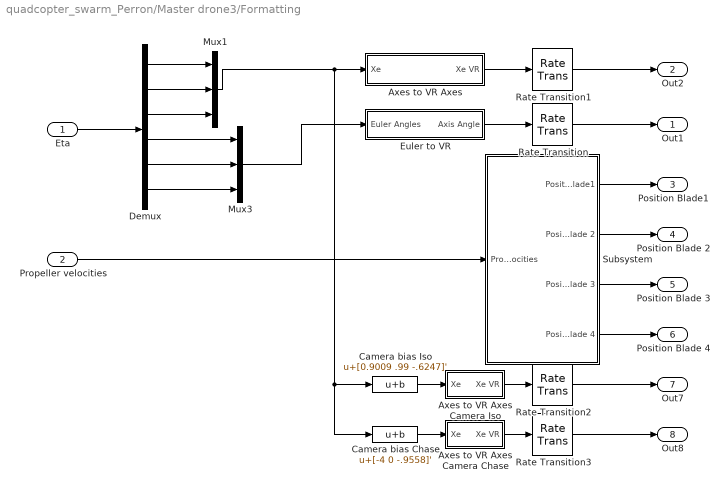
== system quadcopter_swarm_Perron/Master drone3/Formatting ==
  Eta : Inport
  Propeller velocities : Inport  Port=2
  Axes to VR Axes : Subsystem
  Axes to VR Axes Camera Chase : Subsystem
  Axes to VR Axes Camera Iso : Subsystem
  Camera bias Chase : Bias  Bias=[-4 0 -.9558]'  SaturateOnIntegerOverflow=off
  Camera bias Iso : Bias  Bias=[0.9009 .99 -.6247]'  SaturateOnIntegerOverflow=off
  Demux : Demux  Outputs=6
  Euler to VR : Subsystem
  Mux1 : Mux  Inputs=3
  Mux3 : Mux  Inputs=3
  Rate Transition{,1..3} (4 alike) : RateTransition
  Subsystem : Subsystem
  Out1 : Outport
  Out2 : Outport  Port=2
  Position Blade1 : Outport  Port=3
  Position Blade 2 : Outport  Port=4
  Position Blade 3 : Outport  Port=5
  Position Blade 4 : Outport  Port=6
  Out7 : Outport  Port=7
  Out8 : Outport  Port=8
  wires:
  Rate Transition2/1 -> Out7/1
  Propeller velocities/1 -> Subsystem/1(Propeller velocities)
  Subsystem/3(Position Blade 3) -> Position Blade 3/1
  Subsystem/1(Position Blade1) -> Position Blade1/1
  Mux3/1 -> Euler to VR/1(Euler Angles)
  Camera bias Chase/1 -> Axes to VR Axes Camera Chase/1(Xe)
  Axes to VR Axes Camera Chase/1(Xe VR) -> Rate Transition3/1
  Subsystem/2(Position Blade 2) -> Position Blade 2/1
  Axes to VR Axes Camera Iso/1(Xe VR) -> Rate Transition2/1
  Euler to VR/1(Axis Angle) -> Rate Transition/1
  Axes to VR Axes/1(Xe VR) -> Rate Transition1/1
  Rate Transition1/1 -> Out2/1
  Camera bias Iso/1 -> Axes to VR Axes Camera Iso/1(Xe)
  Mux1/1 -> Camera bias Chase/1, Camera bias Iso/1, Axes to VR Axes/1(Xe)
  Rate Transition3/1 -> Out8/1
  Rate Transition/1 -> Out1/1
  Subsystem/4(Position Blade 4) -> Position Blade 4/1
  Demux/2 -> Mux1/2
  Demux/5 -> Mux3/2
  Demux/3 -> Mux1/3
  Eta/1 -> Demux/1
  Demux/1 -> Mux1/1
  Demux/4 -> Mux3/1
  Demux/6 -> Mux3/3

== system quadcopter_swarm_Perron/Master drone3/PID controllers ==
  position ref : Inport
  eta : Inport  Port=2
  Inner-loop controllers : Subsystem
  Manual Switch : ManualSwitch
  Pad3 : dspsigops/Pad  padAlong=Rows  dimsToPad=1  valSrc=Specify via dialog  padVal=0  spec=Output size  padNumOutRowsSpecMethod=User-specified  numOutRows=1  padNumOutColsSpecMethod=User-specified  numOutCols=6  isVarDimsMode=off  padBeginning=0  padEnd=0  outSizeMode=User-specified  outSize=1  padSigAt=Beginning  trunc_flag=None  roundingMode=Floor  overflowMode=off  truncOrWrapMode=Truncate  wrap_flag=None
  Refs (alt. + Euler angles) : Constant  Value=[-20;0;20;0]  VectorParams1D=off
  outer-loop controllers output : Scope
  outer-loop position controller : Subsystem
  tau_p : Outport
  wires:
  position ref/1 -> outer-loop position controller/1(position ref)
  outer-loop position controller/1(alt. + Euler angles) -> Manual Switch/1, outer-loop controllers output/1
  eta/1 -> Inner-loop controllers/2(eta), outer-loop position controller/2(eta_euler)  "eta_euler"
  Refs (alt. + Euler angles)/1 -> Manual Switch/2
  Manual Switch/1 -> Inner-loop controllers/1(refs)  "alt. + Euler angles"
  Pad3/1 -> tau_p/1
  Inner-loop controllers/1(Fz,mx,my,mz) -> Pad3/1

== system quadcopter_swarm_Perron/Master drone3/Quadcopter model Euler ==
  tau_p : Inport
  x_0 : Inport  Port=2
  Gravity : Subsystem
      settings: PortSchema="{\"entries\":[{\"content\":{\"sides\":[{\"content\":{\"connectorIds\":[\"Out1\",\"In1\"]},\"type\":\"ConnectorPlacement.EquallySpacedRectSide\",\"uuid\":\"bc23a1f5-cdb9-4283-9ea4-cdee480fdcbc\"},{\"content\":{\"side\":\"RIGHT\"},\"type\":\"ConnectorPlacement.EquallySpacedRectSide\",\"uuid\":\"6d80009b-5037-4ff5-9c53-c950dec4dc37\"},{\"content\":{\"side\":\"TOP\"},\"type\":\"ConnectorPlacement.EquallySpacedRectSide\",\"uuid\":\"00364382-26ff-4cd9-a2a2-07aec872e2b0\"}]},\"type\":\"ConnectorPlacement.EquallySpacedConnector\",\"uuid\":\"88fcb791-5b95-44c0-bf21-2ced4fb8e0fb\"}],\"packageUris\":[\"http://schema.mathworks.com/mf0/Connector/R2020b\"],\"version\":\"1.0\"}"
  Scope1 : Scope  NumInputPorts=3
  Sum : Sum  Inputs=|++
  kinematics from Euler angles : Subsystem
  rigid-body dynamics : Subsystem
  eta : Outport
  wires:
  kinematics from Euler angles/1(eta) -> eta/1, Gravity/1(eta_euler), Scope1/3
  tau_p/1 -> Sum/1  "tau_p"
  Sum/1 -> Scope1/1, rigid-body dynamics/1(tau)  "tau"
  rigid-body dynamics/1(nu_subsystem) -> Scope1/2, kinematics from Euler angles/1(nu)
  Gravity/1(tau_g) -> Sum/2
  x_0/1 -> kinematics from Euler angles/2(x_0)

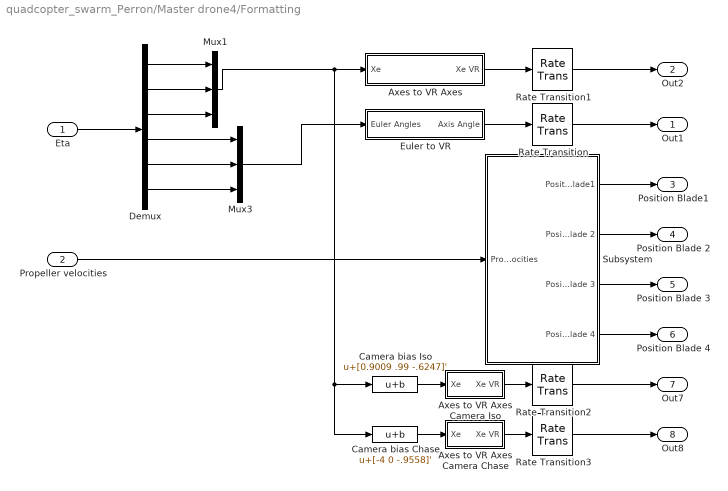
== system quadcopter_swarm_Perron/Master drone4/Formatting ==
  Eta : Inport
  Propeller velocities : Inport  Port=2
  Axes to VR Axes : Subsystem
  Axes to VR Axes Camera Chase : Subsystem
  Axes to VR Axes Camera Iso : Subsystem
  Camera bias Chase : Bias  Bias=[-4 0 -.9558]'  SaturateOnIntegerOverflow=off
  Camera bias Iso : Bias  Bias=[0.9009 .99 -.6247]'  SaturateOnIntegerOverflow=off
  Demux : Demux  Outputs=6
  Euler to VR : Subsystem
  Mux1 : Mux  Inputs=3
  Mux3 : Mux  Inputs=3
  Rate Transition{,1..3} (4 alike) : RateTransition
  Subsystem : Subsystem
  Out1 : Outport
  Out2 : Outport  Port=2
  Position Blade1 : Outport  Port=3
  Position Blade 2 : Outport  Port=4
  Position Blade 3 : Outport  Port=5
  Position Blade 4 : Outport  Port=6
  Out7 : Outport  Port=7
  Out8 : Outport  Port=8
  wires:
  Rate Transition2/1 -> Out7/1
  Propeller velocities/1 -> Subsystem/1(Propeller velocities)
  Subsystem/3(Position Blade 3) -> Position Blade 3/1
  Subsystem/1(Position Blade1) -> Position Blade1/1
  Mux3/1 -> Euler to VR/1(Euler Angles)
  Camera bias Chase/1 -> Axes to VR Axes Camera Chase/1(Xe)
  Axes to VR Axes Camera Chase/1(Xe VR) -> Rate Transition3/1
  Subsystem/2(Position Blade 2) -> Position Blade 2/1
  Axes to VR Axes Camera Iso/1(Xe VR) -> Rate Transition2/1
  Euler to VR/1(Axis Angle) -> Rate Transition/1
  Axes to VR Axes/1(Xe VR) -> Rate Transition1/1
  Rate Transition1/1 -> Out2/1
  Camera bias Iso/1 -> Axes to VR Axes Camera Iso/1(Xe)
  Mux1/1 -> Camera bias Chase/1, Camera bias Iso/1, Axes to VR Axes/1(Xe)
  Rate Transition3/1 -> Out8/1
  Rate Transition/1 -> Out1/1
  Subsystem/4(Position Blade 4) -> Position Blade 4/1
  Demux/2 -> Mux1/2
  Demux/5 -> Mux3/2
  Demux/3 -> Mux1/3
  Eta/1 -> Demux/1
  Demux/1 -> Mux1/1
  Demux/4 -> Mux3/1
  Demux/6 -> Mux3/3

== system quadcopter_swarm_Perron/Master drone4/PID controllers ==
  position ref : Inport
  eta : Inport  Port=2
  Inner-loop controllers : Subsystem
  Manual Switch : ManualSwitch
  Pad3 : dspsigops/Pad  padAlong=Rows  dimsToPad=1  valSrc=Specify via dialog  padVal=0  spec=Output size  padNumOutRowsSpecMethod=User-specified  numOutRows=1  padNumOutColsSpecMethod=User-specified  numOutCols=6  isVarDimsMode=off  padBeginning=0  padEnd=0  outSizeMode=User-specified  outSize=1  padSigAt=Beginning  trunc_flag=None  roundingMode=Floor  overflowMode=off  truncOrWrapMode=Truncate  wrap_flag=None
  Refs (alt. + Euler angles) : Constant  Value=[-20;0;20;0]  VectorParams1D=off
  outer-loop controllers output : Scope
  outer-loop position controller : Subsystem
  tau_p : Outport
  wires:
  position ref/1 -> outer-loop position controller/1(position ref)
  outer-loop position controller/1(alt. + Euler angles) -> Manual Switch/1, outer-loop controllers output/1
  eta/1 -> Inner-loop controllers/2(eta), outer-loop position controller/2(eta_euler)  "eta_euler"
  Refs (alt. + Euler angles)/1 -> Manual Switch/2
  Manual Switch/1 -> Inner-loop controllers/1(refs)  "alt. + Euler angles"
  Pad3/1 -> tau_p/1
  Inner-loop controllers/1(Fz,mx,my,mz) -> Pad3/1

== system quadcopter_swarm_Perron/Master drone4/Quadcopter model Euler ==
  tau_p : Inport
  x_0 : Inport  Port=2
  Gravity : Subsystem
      settings: PortSchema="{\"entries\":[{\"content\":{\"sides\":[{\"content\":{\"connectorIds\":[\"Out1\",\"In1\"]},\"type\":\"ConnectorPlacement.EquallySpacedRectSide\",\"uuid\":\"bc23a1f5-cdb9-4283-9ea4-cdee480fdcbc\"},{\"content\":{\"side\":\"RIGHT\"},\"type\":\"ConnectorPlacement.EquallySpacedRectSide\",\"uuid\":\"6d80009b-5037-4ff5-9c53-c950dec4dc37\"},{\"content\":{\"side\":\"TOP\"},\"type\":\"ConnectorPlacement.EquallySpacedRectSide\",\"uuid\":\"00364382-26ff-4cd9-a2a2-07aec872e2b0\"}]},\"type\":\"ConnectorPlacement.EquallySpacedConnector\",\"uuid\":\"88fcb791-5b95-44c0-bf21-2ced4fb8e0fb\"}],\"packageUris\":[\"http://schema.mathworks.com/mf0/Connector/R2020b\"],\"version\":\"1.0\"}"
  Scope1 : Scope  NumInputPorts=3
  Sum : Sum  Inputs=|++
  kinematics from Euler angles : Subsystem
  rigid-body dynamics : Subsystem
  eta : Outport
  wires:
  kinematics from Euler angles/1(eta) -> eta/1, Gravity/1(eta_euler), Scope1/3
  tau_p/1 -> Sum/1  "tau_p"
  Sum/1 -> Scope1/1, rigid-body dynamics/1(tau)  "tau"
  rigid-body dynamics/1(nu_subsystem) -> Scope1/2, kinematics from Euler angles/1(nu)
  Gravity/1(tau_g) -> Sum/2
  x_0/1 -> kinematics from Euler angles/2(x_0)

== system quadcopter_swarm_Perron/Master drone/Formatting/Axes to VR Axes ==
  Xe : Inport
  Demux : Demux  Outputs=3
      settings: DisplayOption=none
  Mux : Mux  Inputs=3
  rad-->deg1 : Gain  Gain=-1  SaturateOnIntegerOverflow=on  OutDataTypeStr=Inherit: Same as input  ParamDataTypeStr=Inherit: Same as input
  Xe VR : Outport  VectorParamsAs1DForOutWhenUnconnected=off
  wires:
  Xe/1 -> Demux/1
  Demux/1 -> Mux/1
  Demux/3 -> rad-->deg1/1
  Mux/1 -> Xe VR/1
  rad-->deg1/1 -> Mux/2
  Demux/2 -> Mux/3

== system quadcopter_swarm_Perron/Master drone/Formatting/Axes to VR Axes Camera Chase ==
  Xe : Inport
  Demux : Demux  Outputs=3
      settings: DisplayOption=none
  Mux : Mux  Inputs=3
  rad-->deg1 : Gain  Gain=-1  SaturateOnIntegerOverflow=on  OutDataTypeStr=Inherit: Same as input  ParamDataTypeStr=Inherit: Same as input
  Xe VR : Outport  VectorParamsAs1DForOutWhenUnconnected=off
  wires:
  Xe/1 -> Demux/1
  Demux/1 -> Mux/1
  Demux/3 -> rad-->deg1/1
  Mux/1 -> Xe VR/1
  rad-->deg1/1 -> Mux/2
  Demux/2 -> Mux/3

== system quadcopter_swarm_Perron/Master drone/Formatting/Axes to VR Axes Camera Iso ==
  Xe : Inport
  Demux : Demux  Outputs=3
      settings: DisplayOption=none
  Mux : Mux  Inputs=3
  rad-->deg1 : Gain  Gain=-1  SaturateOnIntegerOverflow=on  OutDataTypeStr=Inherit: Same as input  ParamDataTypeStr=Inherit: Same as input
  Xe VR : Outport  VectorParamsAs1DForOutWhenUnconnected=off
  wires:
  Demux/2 -> Mux/3
  rad-->deg1/1 -> Mux/2
  Mux/1 -> Xe VR/1
  Demux/3 -> rad-->deg1/1
  Demux/1 -> Mux/1
  Xe/1 -> Demux/1

== system quadcopter_swarm_Perron/Master drone/Formatting/Euler to VR ==
  Euler Angles : Inport
  Axis Angle Vector : Subsystem
  Mux : Mux  Inputs=2
  Mux1 : Mux  Inputs=2
  Mux2 : Mux  Inputs=2
  Quaternion Multiplication (Pitch & Yaw) : aerolibutil/Quaternion Multiplication
  Quaternion Multiplication (Roll) : aerolibutil/Quaternion Multiplication
  Quaternion Normalization : Subsystem
  Quaternion Normalization1 : Subsystem
  Quaternion Normalization2 : Subsystem
  Selector : Selector  InputPortWidth=3  IndexOptions=Index vector (dialog)  Indices=[3]  OutputSizes=1
  Selector1 : Selector  InputPortWidth=3  IndexOptions=Index vector (dialog)  Indices=[2]  OutputSizes=1
  Selector2 : Selector  InputPortWidth=3  IndexOptions=Index vector (dialog)  Indices=[1]  OutputSizes=1
  Vr Pitch Axes : Constant  Value=[0 0 1]
  Vr Roll Axes : Constant  Value=[1 0 0]
  Vr Yaw Axes : Constant  Value=[0 -1 0]
  Axis Angle : Outport  VectorParamsAs1DForOutWhenUnconnected=off
  wires:
  Quaternion Multiplication (Roll)/1 -> Axis Angle Vector/1(e0)
  Axis Angle Vector/1(e0_norm) -> Axis Angle/1
  Quaternion Normalization/1(e0_norm) -> Quaternion Multiplication (Roll)/2
  Quaternion Normalization2/1(e0_norm) -> Quaternion Multiplication (Pitch & Yaw)/1
  Quaternion Normalization1/1(e0_norm) -> Quaternion Multiplication (Pitch & Yaw)/2
  Mux2/1 -> Quaternion Normalization2/1(e0)
  Mux1/1 -> Quaternion Normalization1/1(e0)
  Mux/1 -> Quaternion Normalization/1(e0)
  Selector/1 -> Mux2/1
  Vr Yaw Axes/1 -> Mux2/2
  Selector1/1 -> Mux1/1
  Vr Pitch Axes/1 -> Mux1/2
  Selector2/1 -> Mux/1
  Vr Roll Axes/1 -> Mux/2
  Euler Angles/1 -> Selector2/1, Selector1/1, Selector/1
  Quaternion Multiplication (Pitch & Yaw)/1 -> Quaternion Multiplication (Roll)/1

== system quadcopter_swarm_Perron/Master drone/Formatting/Subsystem ==
  Propeller velocities : Inport
  Bias : Bias  Bias=.1  SaturateOnIntegerOverflow=off
  Bias1 : Bias  Bias=-.3  SaturateOnIntegerOverflow=off
  Bias2 : Bias  Bias=.5  SaturateOnIntegerOverflow=off
  Bias3 : Bias  Bias=.7  SaturateOnIntegerOverflow=off
  Constant : Constant  Value=[0 1 0]
  Data Type Conversion : DataTypeConversion  OutDataTypeStr=double  SaturateOnIntegerOverflow=off  RndMeth=Floor
  Demux : Demux
  Gain : Gain  Gain=1.38408
  Integrator : Integrator  InitialCondition=[.1 ; .2 ;-.3 ;-.4]  WrapState=on  WrappedStateUpperValue=2*pi  WrappedStateLowerValue=-2*pi
  Mux{,1..3} (4 alike) : Mux  Inputs=2
  Rate Transition2 : RateTransition
  Position Blade1 : Outport  VectorParamsAs1DForOutWhenUnconnected=off
  Position Blade 2 : Outport  Port=2  VectorParamsAs1DForOutWhenUnconnected=off
  Position Blade 3 : Outport  Port=3  VectorParamsAs1DForOutWhenUnconnected=off
  Position Blade 4 : Outport  Port=4  VectorParamsAs1DForOutWhenUnconnected=off
  wires:
  Bias3/1 -> Mux3/2
  Mux3/1 -> Position Blade 4/1
  Bias1/1 -> Mux1/2
  Bias2/1 -> Mux2/2
  Demux/2 -> Bias1/1
  Constant/1 -> Mux3/1, Mux2/1, Mux1/1, Mux/1
  Mux1/1 -> Position Blade 2/1
  Mux2/1 -> Position Blade 3/1
  Integrator/1 -> Rate Transition2/1
  Mux/1 -> Position Blade1/1
  Demux/3 -> Bias2/1
  Bias/1 -> Mux/2
  Propeller velocities/1 -> Data Type Conversion/1
  Demux/4 -> Bias3/1
  Rate Transition2/1 -> Demux/1
  Demux/1 -> Bias/1
  Data Type Conversion/1 -> Gain/1
  Gain/1 -> Integrator/1
